simulink model "Sim7_test_var_load"  (R2018a)
settings: Solver=ode1  StartTime=0.0  StopTime=10  FixedStep=Time_Step  MaxStep=1e-4  RelTol=1e-3
undefined symbols (not defined in the file): Bxx_GenericVoltageSource, Lg, Rg, Source_Lib, Theta0, Time_Step, Ug, Un, V0, VSC01_id0
libraries: powerlib x29, Control_Lib x5, simulink x4
(part 1 of 2)
settings Model: Creator=Frederic_Colas  LastModifiedBy=fcolas
settings OptimizationCC: LifeSpan=inf
settings DebuggingCC: UnconnectedInputMsg=none  UnconnectedOutputMsg=none  UnconnectedLineMsg=none  SFExecutionAtInitializationDiag=none
settings HardwareCC: ProdBitPerSizeT=32  ProdBitPerPtrDiffT=32  ProdWordSize=32  ProdHWDeviceType=Specified
settings CodeAppCC: StateflowObjectComments=on
settings SimscapeCC: SimscapeNormalizeSystem=off

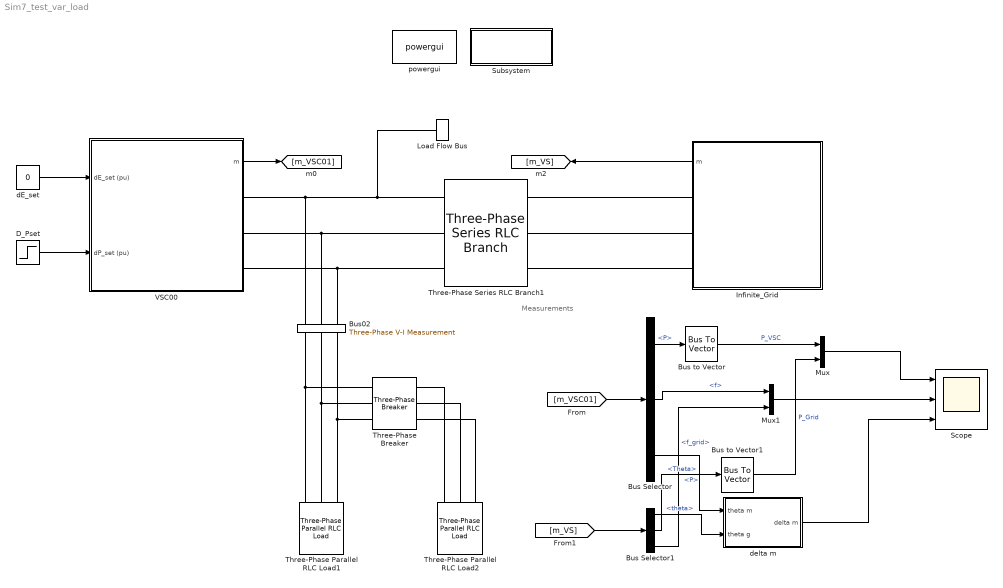
== system Sim7_test_var_load ==
  note: Measurements
  Bus Selector : BusSelector  OutputSignals=P,f,Theta.Theta
  Bus Selector1 : BusSelector  OutputSignals=Theta.theta,P,f_grid
  Bus to Vector : BusToVector
  Bus to Vector1 : BusToVector
  "Bus02 " : powerlib/Measurements/Three-Phase V-I Measurement  VoltageMeasurement=no  SetLabelV=off  LabelV=Vabc  Vpu=off  VpuLL=off  CurrentMeasurement=no  SetLabelI=off  LabelI=Iabc  Ipu=off  Pbase=100e6  Vbase=500e3  OutputType=Complex  PhasorSimulation=off  PSBequivalent=0
  D_Pset : Step  After=0  SampleTime=0
  Infinite_Grid : Subsystem  AncestorBlock=Source_Lib/Bxx_GenericVoltageSource  mask(GenericVoltageSource){SourceNature_str=INERTIAL, fn=50, Sn=1e9, Un=Un, LFpopup=Swing, P0=149805764.7076, Q0=1121677.2891, V0_pu=1, U0=20000, Theta0_deg=0, H_s=5, DroopOnOff=on, R_percent=4, TN=1, TD=2}
      mask prompts: SourceNature_str "Nature of the voltage source"; fn "Nominal frequency fn [Hz]"; Sn "Nominal apparent power Sn [VA]"; Un "Nominal voltage Un [V RMS Ph2Ph]"; P0 "Active power P0 [W]"; Q0 "Reactive power Q0 [VAR]"; V0_pu "Initial pu voltage V0_pu [pu]"; U0 "Initial voltage U0 [Vrms Ph2Ph]"; Theta0_deg "Initial angle (°)"; H_s "Inertia H [s]"; DroopOnOff "Frequency DROOP activation"; R_percent "Droop gain Kp [%]"; TN "Network time constant Lead [s]"; TD "Network time constant Lag [s]"
      mask init:
      | % Update Name of LF bus for internal purpose
      | NameStr = [get_param(gcb,'Name')];% '_LF'];
      | set_param([gcb '/Load Flow Bus'],'ID',NameStr);  
      | 
      | % Base specification
      | fb = fn;                % [Hz] base frequency
      | Sb = Sn;                % [VA] base power
      | Ub = Un;                % [V] base ph2ph voltage
      | Vb = Un/sqrt(3);        % [V] base ph2N voltage
      | Ib = Sb/(3*Vb);         % [A] base current
      | Zb = Vb*Ib;             % [Ohm] base impedance
      | 
      | % Set the frequency droop gain
      | R = R_percent / 100;
      | 
      | %Initialize correctly the LoadFlow bus parameters connected to PCC
      |     VLF = V0_pu;
      |     ThetaLF = Theta0_deg;
      |     if (LFpopup == 'PQ')
      |         VLF = 1;
      |         ThetaLF = 0;
      |     elseif (LFpopup == 'PV')
      |         VLF = V0_pu;
      |         ThetaLF = 0;        
      |     end
      |     set_param([gcb '/Load Flow Bus'],'Vref',num2str(VLF),'Vangle',num2str(ThetaLF));
      | 
      | 
      | % Update mask display:
      | % mo = get_param(gcb,'MaskObject');
      mask TypeOptions SourceNature_str: INFINITE | INERTIAL
      mask Callback SourceNature_str:
      | % Get the mask parameter values. This is a cell
      | %   array of character vectors.
      | maskStr = get_param(gcb,'SourceNature_str');
      | p=Simulink.Mask.get(gcb);
      | 
      | % The pop-up menu is the first mask parameter.
      | %   Check the value selected in the pop-up
      | if strcmp(maskStr,'INFINITE')
      |    p.getParameter('H_s').Visible='off';
      |    p.getParameter('DroopOnOff').Visible='off';
      |    DroopOnOff = 'off';
      |    p.getParameter('R_percent').Visible='off';
      |    p.getParameter('TN').Visible='off';
      |    p.getParameter('TD').Visible='off';
      |    set_param([gcb '/SourceNature'],'Value','1')
      | else
      |    p.getParameter('H_s').Visible='on';
      |    p.getParameter('DroopOnOff').Visible='on';
      |    DroopOnOff = 'on';
      |    p.getParameter('R_percent').Visible='on';
      |    p.getParameter('TN').Visible='on';
      |    p.getParameter('TD').Visible='on';
      |    set_param([gcb '/SourceNature'],'Value','2')
      | end
      mask TypeOptions LFpopup: Swing | PQ | PV
      mask Callback LFpopup:
      | % Get the mask parameter values. This is a cell
      | %   array of character vectors.
      | maskStr = get_param(gcb,'LFpopup');
      | p=Simulink.Mask.get(gcb);
      | 
      | % The pop-up menu is the first mask parameter.
      | %   Check the value selected in the pop-up
      | if strcmp(maskStr,'Swing'),
      | 
      |     % Set the visibility of both parameters on when
      |     %   User-defined is selected in the pop-up.
      |     p.getParameter('P0').Enabled='off';
      |     p.getParameter('Q0').Enabled='off';
      |     p.getParameter('V0_pu').Enabled='on';
      |     p.getParameter('U0').Enabled='off';
      |     p.getParameter('Theta0_deg').Enabled='off';
      |     set_param([gcb '/Source_For_LF'],'BusType','swing');
      | 
      | elseif strcmp(maskStr,'PQ'),
      | 
      |     % Set the visibility of both parameters on when
      |     %   User-defined is selected in the pop-up.
      |     p.getParameter('P0').Enabled='on';
      |     p.getParameter('Q0').Enabled='on';
      |     p.getParameter('V0_pu').Enabled='off';
      |     p.getParameter('U0').Enabled='off';
      |     p.getParameter('Theta0_deg').Enabled='off';
      |     set_param([gcb '/Source_For_LF'],'BusType','PQ');
      | 
      |     % Turn off the visibility of the Value field
      |     %   when User-defined is not selected.
      | else
      | 
      |     % Set the visibility of both parameters on when
      |     %   User-defined is selected in the pop-up.
      |     p.getParameter('P0').Enabled='on';
      |     p.getParameter('Q0').Enabled='off';
      |     p.getParameter('V0_pu').Enabled='on';
      |     p.getParameter('U0').Enabled='off';
      |     p.getParameter('Theta0_deg').Enabled='off';
      |     set_param([gcb '/Source_For_LF'],'BusType','PV');
      | 
      | end
      mask Callback DroopOnOff:
      | % Get the mask parameter values. This is a cell
      | %   array of character vectors.
      | maskStr = get_param(gcb,'DroopOnOff');
      | p=Simulink.Mask.get(gcb);
      | 
      | if strcmp(maskStr,'on'),
      |     p.getParameter('R_percent').Enabled='on';
      | else
      |     p.getParameter('R_percent').Enabled='off';
      | end
      mask DialogControl Container2 Prompt: Nominal specification (for base definition)
      mask DialogControl Container3 Prompt: Loadflow specification
      mask DialogControl InertialConfig Prompt: Inertial source configuration
  Load Flow Bus : powerlib/Measurements/Load Flow Bus  LConnTagsString=a  Phases=single  Connectors=on one side  ID=BUS_1  Vbase=Un  Vref=1  Vangle=0  VLF=0.9992  VLFb=1  VLFc=1  angleLF=-0.4292  angleLFb=0  angleLFc=0
  Mux : Mux  Inputs=2
  Mux1 : Mux  Inputs=2
  Scope : Scope  NumInputPorts=3
  Subsystem : Subsystem
      settings: OpenFcn=LoadFlow_VSC
      mask Display: color('blue'),disp('Update Loadflow')
  Three-Phase Parallel RLC Load1 : powerlib/Elements/Three-Phase Parallel RLC Load  LConnTagsString=A|B|C  Configuration=Y (grounded)  NominalVoltage=Ug  Vabc=[1e3 1e3 1e3]  Vabcp=[1e3 1e3 1e3]  NominalFrequency=fb  UnbalancedPower=off  ActivePower=300e6  InductivePower=0  CapacitivePower=0  Pabc=[10e3 9e3 11e3]  QLabc=[100 90 110]  QCabc=[100 90 110]  Pabcp=[10e3 9e3 11e3]  QLabcp=[100 90 110]  QCabcp=[100 90 110]  Measurements=None  LoadType=constant Z
  Three-Phase Parallel RLC Load2 : powerlib/Elements/Three-Phase Parallel RLC Load  LConnTagsString=A|B|C  Configuration=Y (grounded)  NominalVoltage=Ug  Vabc=[1e3 1e3 1e3]  Vabcp=[1e3 1e3 1e3]  NominalFrequency=fb  UnbalancedPower=off  ActivePower=500e6  InductivePower=0  CapacitivePower=0  Pabc=[10e3 9e3 11e3]  QLabc=[100 90 110]  QCabc=[100 90 110]  Pabcp=[10e3 9e3 11e3]  QLabcp=[100 90 110]  QCabcp=[100 90 110]  Measurements=None  LoadType=constant Z
  Three-Phase Series RLC Branch1 : powerlib/Elements/Three-Phase Series RLC Branch  LConnTagsString=A|B|C  RConnTagsString=A|B|C  BranchType=RL  Resistance=Rg  Inductance=Lg  Capacitance=1e-6  Measurements=None
  Three-Phase Breaker : powerlib/Elements/Three-Phase Breaker  InitialState=open  SwitchA=on  SwitchB=on  SwitchC=on  SwitchTimes=0.5  External=off  BreakerResistance=0.01  SnubberResistance=1e6  SnubberCapacitance=inf  Measurements=None
  VSC00 : Subsystem  mask(VSC){fn=50, Sn=1000e6, Pn=1000e6, Udcn=640e3, Time_Step=Time_Step, Un1=320e3, Un2=Ug, Rt_pu=0.005, Lt_pu=0.15, Lm_pu=500, Rm_pu=500, Tr_PLL=10, Val_Freq_Support=off, R_percent=4, Rv=0.09, W_TVR=60, I_max_VI_pu=1.2, DX_DR=5, Val_Mod_H=off, I_max_pu=1.25, Tr_I_max=200, Advanced=off, gainpopup=With Inertia, f_Inertia_Less=5/(2*pi), zeta_Inertia_Less=1, Param_Inertia=PI, H_GFo=5, zeta_GFo=0.7, LFpopup=PQ, P0=0.15, Q0=2.3716e-08, V0=0.99922, Theta0=-0.42918}
      mask prompts: fn "Nominal Frequency (Hz)"; Sn "Nominal Apparent Power (VA)"; Pn "Nominal Power (W)"; Udcn "Nominal DC Voltage (V)"; Time_Step "Sample Time (s)"; Un1 "VSC side Nominal Ph-Ph Voltage (V)"; Un2 "Grid side Nominal Ph-Ph Voltage (V)"; Rt_pu "R (pu)"; Lt_pu "L (pu)"; Lm_pu "Rm (pu)"; Rm_pu "Lm (pu)"; Tr_PLL "Time response (ms)"; Val_Freq_Support "Frequency Support"; R_percent "Droop Gain (%)"; Rv "Damping Resistance (Rv)"; W_TVR "Dr filter"; I_max_VI_pu "Current Threshold (pu)"; Val_Mod_H "Inertia Modulation"; I_max_pu "I max (pu)"; Tr_I_max "Current Loop time response (ms)"; gainpopup "Strategy"; f_Inertia_Less "Bandwidth (Hz)"; zeta_Inertia_Less "Damping"; H_GFo "Inertia H (s)"; zeta_GFo "Damping Ratio"; P0 "Initial Active Power (pu)"; Q0 "Initial Reactive Power (pu)"; V0 "Initial Voltage (pu)"; Theta0 "Initial Angle (°)"
      mask init:
      | % Update Name of LF bus for internal purpose
      |     %NameStr = [get_param(gcb,'Name')];% '_LF'];
      |     %set_param([gcb '/Load Flow Bus'],'ID',NameStr);    
      |     
      | % Base values
      |     fb = fn;
      |     Pb = Pn;
      |     cos_phi_n = Pn/Sn;
      |     Sb = Pb/cos_phi_n;
      |     Vn1 = Un1/sqrt(3);
      |     Vb1 = Vn1;
      |     Vn2 = Un2/sqrt(3);
      |     Vb2 = Vn2;
      |     Ib1 = Sb / 3*Vb1;
      |     Ib2 = Sb / (3*Vb2);
      |     wb = 2*pi*fb;
      |   
      | % PLL derivation of the parameters
      |     wn_PLL=5/Tr_PLL;
      |     zeta_PLL = 1;
      |     Kp_PLL_pu = 2*zeta_PLL*wn_PLL/wb;
      |     Ki_PLL_pu = wn_PLL^2/wb;
      |     
      | % Grid-Forming control tuning
      |     % Inertia Less
      |     wn_Inertia_Less = 2*pi*f_Inertia_Less;
      |     Ki_Inertia_Less = Lt_pu*wn_Inertia_Less^2/wb;
      |     Kp_Inertia_Less = 2*zeta_Inertia_Less*wn_Inertia_Less*Lt_pu/wb;
      |     
      |     % With Inertia
      |     Kc = 1/(Lt_pu);
      |     kp_GFo = zeta_GFo*sqrt(2/(H_GFo*wb*Kc));
      |     kd = 2*H_GFo*kp_GFo*Kc*wb;
      | 
      | % Virtual Impedance tuning
      |     X_VI = roots([1/DX_DR^2+1 2*Lt_pu Lt_pu^2-1/I_max_VI_pu^2]);
      |     X_VI = max(X_VI);
      |     Kp_Rvi_pu = X_VI/(DX_DR*(I_max_VI_pu-1)); 
      |     
      | % Set the chosen strategy
      |     if (gainpopup == 1)
      |         Chosen_Strategy = 1;
      |     elseif (gainpopup == 2)
      |         if (Param_Inertia == 1)
      |             Chosen_Strategy = 2;
      |         elseif (Param_Inertia == 2)
      |             Chosen_Strategy = 3;
      |         end
      |     end
      |     
      | % Set the frequency droop gain
      |     R = R_percent / 100;
      | 
      | % Compute the delay compensation between control and power parts
      |     if (Time_Step == -1)
      |         Solver_Time_Step = 0;
      |     else
      |         Solver_Time_Step = Time_Step;
      |     end
      | 
      | % Compute Initial Voltage of VSC 
      | %   from steady-state output transformer model and Loadflow result
      |     
      |     %Initialize correctly the LoadFlow bus parameters connected to PCC
      |     VLF = V0;
      |     ThetaLF = Theta0;
      |     %if (LFpopup == 'PQ')
      |     %    VLF = 1;
      |     %    ThetaLF = 0;
      |     %elseif (LFpopup == 'PV')
      |     %%    VLF = V0;
      |     %    ThetaLF = 0;        
      |     %end
      |     %set_param([gcb '/Load Flow Bus'],'Vref',num2str(VLF),'Vangle',num2str(ThetaLF));
      |     
      |     R1_pu = Rt_pu/2;
      |     L1_pu = Lt_pu/2;
      |     R2_pu = Rt_pu/2;
      |     L2_pu = Lt_pu/2;
      |     X1_pu = L1_pu;
      |     X2_pu = L2_pu;
      |     Xm_pu = Lm_pu;
      |     
      |     Zm_pu = 1/(1/Rm_pu+1/(1i*Xm_pu));
      | 
      |     S0=P0+1i*Q0;
      |     I2 = conj(S0)/(V0);
      | 
      |     Vm = (R2_pu+1i*X2_pu)*I2 + V0;
      |     Im = Vm/Zm_pu;
      | 
      |     I1 = I2 + Im;
      |     V1 = (R1_pu+1i*X1_pu) * I1 + Vm;
      | 
      |     Vvsc0 = abs(V1);
      |     Theta_vsc0 = angle(V1) * 180/pi+Theta0;
      |     
      |     Va0 = Vvsc0*sqrt(2)*Vb1*sin(Theta_vsc0*pi/180);
      |     Vb0 = Vvsc0*sqrt(2)*Vb1*sin(Theta_vsc0*pi/180-2*pi/3);
      |     Vc0 = Vvsc0*sqrt(2)*Vb1*sin(Theta_vsc0*pi/180+2*pi/3);
      |     
      | % Generate string to display LF results on Mask
      |     %str_tmp = fprintf("Vvsc0 = %d, Theta_vsc0 = %d°",Vvsc0,Theta_vsc0);
      |     mo = get_param(gcb,'MaskObject');
      |     mo.getDialogControl('LF_vsc_str').Prompt = ['V0 = ', num2str(Vvsc0),' pu, Angle = ', num2str(Theta_vsc0),'°'];
      |     mo.getDialogControl('LF_pcc_str').Prompt = ['V0 = ', num2str(V0),' pu, Angle = ', num2str(Theta0),'°'];
      |     mo.getDialogControl('LF_pcc_Power_str').Prompt = ['P0 = ', num2str(P0),' pu, Q0 = ', num2str(Q0),' pu'];
      |     %set_param([gcb],'LF_str',str_tmp);
      settings: OpenFcn=|
      | NameStr = get_param(gcb,'Name');
      | open_system(gcbh, 'Mask');
      | 
      | h2AllOpenDlgs = DAStudio.ToolRoot.getOpenDialogs;
      | 
      | for i=1:length(h2AllOpenDlgs)
      |     try
      |          %disp(h2AllOpenDlgs(i).getSource.getBlock.Name);
      |         Dialog_block_name = h2AllOpenDlgs(i).getSource.getBlock.Name;
      |          %strcmp(Dialog_block_name, NameStr),
      |         if (strcmp(h2AllOpenDlgs(i).getSource.getBlock.Name, NameStr))
      |             iPos = h2AllOpenDlgs(i).position;
      |             h2AllOpenDlgs(i).position = [iPos(1)   iPos(2)   iPos(3)*1.4   iPos(4)];
      |         end
      |     end
      | end
      mask Callback Advanced:
      | % Get the mask parameter values. This is a cell
      | %   array of character vectors.
      | maskStr = get_param(gcb,'Advanced');
      | p=Simulink.Mask.get(gcb);
      | 
      | % The pop-up menu is the first mask parameter.
      | %   Check the value selected in the pop-up
      | if strcmp(maskStr,'on'),
      | 
      |     % Set the visibility of both parameters on when
      |     %   User-defined is selected in the pop-up.
      |     p.getDialogControl('TVR').Visible='on';
      |     p.getDialogControl('TVI').Visible='on';
      |     %p.getDialogControl('LC_Filter').Visible='on';
      |     p.getDialogControl('Current_Sat').Visible='on';
      |     %p.getDialogControl('Param_Strat_3').Visible='off';
      | 
      | 
      | else
      | 
      |     % Set the visibility of both parameters on when
      |     %   User-defined is selected in the pop-up.
      |     p.getDialogControl('TVR').Visible='off';
      |     p.getDialogControl('TVI').Visible='off';
      |     %p.getDialogControl('LC_Filter').Visible='off';
      |     p.getDialogControl('Current_Sat').Visible='off';
      |     %p.getDialogControl('Param_Strat_3').Visible='off';
      | 
      | end
      mask TypeOptions gainpopup: Inertia Less | With Inertia
      mask Callback gainpopup:
      | % Get the mask parameter values. This is a cell
      | %   array of character vectors.
      | maskStr = get_param(gcb,'gainpopup');
      | p=Simulink.Mask.get(gcb);
      | 
      | % The pop-up menu is the first mask parameter.
      | %   Check the value selected in the pop-up
      | if strcmp(maskStr,'Inertia Less'),
      | 
      |     % Set the visibility of both parameters on when
      |     %   User-defined is selected in the pop-up.
      |     p.getDialogControl('No_Inertia').Visible='on';
      |     p.getDialogControl('Inertia').Visible='off';
      |     %p.getDialogControl('Param_Strat_3').Visible='off';
      | 
      | 
      | elseif strcmp(maskStr,'With Inertia'),
      | 
      |     % Set the visibility of both parameters on when
      |     %   User-defined is selected in the pop-up.
      |     p.getDialogControl('No_Inertia').Visible='off';
      |     p.getDialogControl('Inertia').Visible='on';
      |     %p.getDialogControl('Param_Strat_3').Visible='off';
      | 
      | 
      |     % Turn off the visibility of the Value field
      |     %   when User-defined is not selected.
      | 
      | else
      | 
      |     % Set the visibility of both parameters on when
      |     %   User-defined is selected in the pop-up.
      |     p.getDialogControl('No_Inertia').Visible='off';
      |     p.getDialogControl('Inertia').Visible='off';
      |     %p.getDialogControl('Param_Strat_3').Visible='off';
      | 
      | end
      mask TypeOptions Param_Inertia: VSM | PI
      mask TypeOptions LFpopup: Swing | PQ | PV
      mask Callback LFpopup:
      | % Get the mask parameter values. This is a cell
      | %   array of character vectors.
      | maskStr = get_param(gcb,'LFpopup');
      | p=Simulink.Mask.get(gcb);
      | 
      | % The pop-up menu is the first mask parameter.
      | %   Check the value selected in the pop-up
      | if strcmp(maskStr,'Swing'),
      | 
      |     % Set the visibility of both parameters on when
      |     %   User-defined is selected in the pop-up.
      |     p.getParameter('P0').Visible='off';
      |     p.getParameter('Q0').Visible='off';
      |     p.getParameter('V0').Visible='on';
      |     p.getParameter('Theta0').Visible='on';
      |     set_param([gcb '/Source_For_LF'],'BusType','swing');
      | 
      | elseif strcmp(maskStr,'PQ'),
      | 
      |     % Set the visibility of both parameters on when
      |     %   User-defined is selected in the pop-up.
      |     p.getParameter('P0').Visible='on';
      |     p.getParameter('Q0').Visible='on';
      |     p.getParameter('V0').Visible='off';
      |     p.getParameter('Theta0').Visible='off';
      |     set_param([gcb '/Source_For_LF'],'BusType','PQ');
      | 
      |     % Turn off the visibility of the Value field
      |     %   when User-defined is not selected.
      | else
      | 
      |     % Set the visibility of both parameters on when
      |     %   User-defined is selected in the pop-up.
      |     p.getParameter('P0').Visible='on';
      |     p.getParameter('Q0').Visible='off';
      |     p.getParameter('V0').Visible='on';
      |     p.getParameter('Theta0').Visible='off';
      |     set_param([gcb '/Source_For_LF'],'BusType','PV');
      | 
      | end
      mask DialogControl Nominal_Param Prompt: Nominal Value
      mask DialogControl Container20 Prompt: Passive Components
      mask DialogControl Control_Param Prompt: Control Parameter
      mask DialogControl Container13 Prompt: PLL
      mask DialogControl Container14 Prompt: Frequency Support
      mask DialogControl TVR Prompt: Transient Virtual Resistor
      mask DialogControl TVI Prompt: Virtual Impedance
      mask DialogControl Current_Sat Prompt: Current Limitation
      mask DialogControl Container18 Prompt: Control Strategy
      mask DialogControl LF_Param Prompt: Loadflow
      mask DialogControl Control4 Prompt: Initial Operating Point
      mask DialogControl Container24 Prompt: VSC side
      mask DialogControl LF_vsc_str Prompt: V0 = 1.0004 pu, Angle = 0.869°
      mask DialogControl Container25 Prompt: PCC
      mask DialogControl LF_pcc_str Prompt: V0 = 0.99922 pu, Angle = -0.42918°
      mask DialogControl LF_pcc_Power_str Prompt: P0 = 0.15 pu, Q0 = 2.3716e-08 pu
      mask DialogControl UpdateLoadflow Prompt: Update Loadflow
      mask DialogControl UpdateLoadflow Callback: LoadFlow_VSC
      mask Display:
      | x1=0.05;
      | y1=0.2;
      | %
      | plot([0.5 0.5]+x1,[0.97,0.8]-y1)
      | plot([0.5 0.32]+x1,[0.80 0.71]-y1)
      | plot([0.32 0.32]+x1,[0.80 0.52]-y1)
      | plot([0.32 0.5]+x1,[0.62 0.52]-y1)
      | plot([0.5 0.5]+x1,[0.52 0.35]-y1)
      | plot([0.45 0.5 0.43]+x1,[0.59 0.52 0.51]-y1)
      | %
      | plot([0.28 0.28]+x1,[0.74 0.58]-y1)
      | plot([0.28 0.20]+x1,[0.66 0.66]-y1)
      | %
      | plot([0.5 0.63]+x1,[0.84 0.84]-y1)
      | plot([0.63 0.63]+x1,[0.84 0.72]-y1)
      | plot([0.63 0.59]+x1,[0.72 0.65]-y1)
      | plot([0.63 0.67]+x1,[0.72 0.65]-y1)
      | plot([0.59 0.67]+x1,[0.65 0.65]-y1)
      | plot([0.63 0.63]+x1,[0.65 0.47]-y1)
      | plot([0.5 0.63]+x1,[0.47 0.47]-y1)
      | plot([0.58 0.67]+x1,[0.72 0.72]-y1)
      | %
      | color('blue')
      | text(0.3,0.10,'L-Filter GFo')
      | port_label('input',1,'dE_set (pu)');
      | port_label('input',2,'dP_set (pu)');
      | port_label('output',1,'m');
      | port_label('rconn',1,'A');
      | port_label('rconn',2,'B');
      | port_label('rconn',3,'C');
  dE_set : Constant  Value=0
  delta m : Subsystem
  powergui : powerlib/powergui  Priority=1  SimulationMode=Discrete  SampleTime=Time_Step  frequency=60  Iterations=50  frequencyindice=50  Pbase=1000000000  ErrMax=1e-6  UnitsV=kV  UnitsW=MW  buscounter=0  FunctionMessages=off  echomessages=off  EnableUseOfTLC=off  CurrentSourceSwitches=off  DisableSnubberDevices=off  DisableRonSwitches=off  DisableVfSwitches=off  DisplayEquations=off  AutomaticDiscreteSolvers=off  SolverType=Tustin/Backward Euler (TBE)  Interpol=off  ExternalGateDelay=off  methode=off  Ts=100  x0status=blocks  SPID=on  SwTol=0  HookPort=off  NonlinearTolerance=1e-4  nMaxIteration=100  ContinueOnMaxIteration=off  RestoreLinks=warning  ResistiveCurrentMeasurement=off  Frange=[0:2:500]  Ylog=off  Xlog=on  ShowGrid=off  save=off  variable=ZData  structure=0  ZoomFFT=off  StartTime=0.0  cycles=1  DisplayStyle=1  fundamental=60  FreqAxis=off  MaxFrequency=1000  frequencyindicesteady=1  RmsSteady=1  display=off
  wires:
  dE_set/1 -> VSC00/1(dE_set (pu))
  D_Pset/1 -> VSC00/2(dP_set (pu))
  VSC00/1(m) -> [m_VSC01]
  Infinite_Grid/1(m) -> [m_VS]
  Bus Selector1/1 -> delta m/2(theta g)  "<theta>"
  Bus Selector/2 -> Mux1/1  "<f>"
  [m_VSC01] -> Bus Selector/1
  [m_VS] -> Bus Selector1/1
  Bus Selector/3 -> delta m/1(theta m)  "<Theta>"
  Bus Selector1/2 -> Bus to Vector1/1  "<P>"
  Mux/1 -> Scope/1
  Mux1/1 -> Scope/2
  Bus Selector/1 -> Bus to Vector/1  "<P>"
  Bus Selector1/3 -> Mux1/2  "<f_grid>"
  Bus to Vector/1 -> Mux/1  "P_VSC"
  Bus to Vector1/1 -> Mux/2  "P_Grid"
  delta m/1(delta m) -> Scope/3
  connections:
  VSC00/RConn1 -- "Bus02 "/LConn3 -- Load Flow Bus/LConn1 -- Three-Phase Series RLC Branch1/LConn1
  VSC00/RConn3 -- "Bus02 "/LConn1 -- Three-Phase Series RLC Branch1/LConn3
  VSC00/RConn2 -- "Bus02 "/LConn2 -- Three-Phase Series RLC Branch1/LConn2
  Infinite_Grid/RConn1 -- Three-Phase Series RLC Branch1/RConn1
  Infinite_Grid/RConn2 -- Three-Phase Series RLC Branch1/RConn2
  Infinite_Grid/RConn3 -- Three-Phase Series RLC Branch1/RConn3
  Three-Phase Breaker/LConn2 -- Three-Phase Parallel RLC Load1/LConn2 -- "Bus02 "/RConn2
  Three-Phase Breaker/LConn1 -- Three-Phase Parallel RLC Load1/LConn1 -- "Bus02 "/RConn3
  Three-Phase Breaker/LConn3 -- Three-Phase Parallel RLC Load1/LConn3 -- "Bus02 "/RConn1
  Three-Phase Parallel RLC Load2/LConn3 -- Three-Phase Breaker/RConn3
  Three-Phase Parallel RLC Load2/LConn2 -- Three-Phase Breaker/RConn2
  Three-Phase Breaker/RConn1 -- Three-Phase Parallel RLC Load2/LConn1

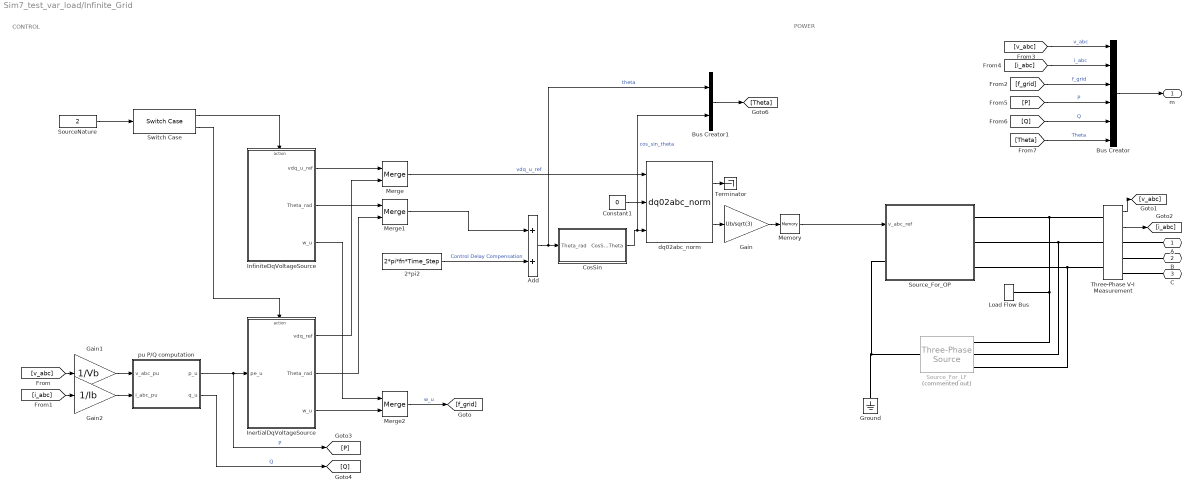
== system Sim7_test_var_load/Infinite_Grid ==
  note: POWER
  note: CONTROL
  " pu P/Q computation" : Subsystem  DialogController=POWERSYS.PowerSysDialog
  2*pi2 : Constant  Value=2*pi*fn*Time_Step
  Add : Sum
  Bus Creator : BusCreator  Inputs=6
  Bus Creator1 : BusCreator  Inputs=2
  Constant1 : Constant  Value=0
  CosSin : Subsystem
  Gain : Gain  Gain=Ub/sqrt(3)
  Gain1 : Gain  Gain=1/Vb
  Gain2 : Gain  Gain=1/Ib
  Ground : powerlib/Elements/Ground  LConnTagsString=a
  InertialDqVoltageSource : Subsystem  TreatAsAtomicUnit=on
  InfiniteDqVoltageSource : Subsystem  TreatAsAtomicUnit=on
  Load Flow Bus : powerlib/Measurements/Load Flow Bus  LConnTagsString=a  Phases=single  Connectors=on one side  ID=Infinite_Grid  Vbase=Un  Vref=1  Vangle=0  VLF=1  VLFb=1  VLFc=1  angleLF=0  angleLFb=0  angleLFc=0
  Memory : Memory
  Merge : Merge
  Merge1 : Merge
  Merge2 : Merge
  SourceNature : Constant  Value=2
  Source_For_LF : powerlib/Electrical Sources/Three-Phase Source  Commented=on  InternalConnection=Yn  VoltagePhases=off  Voltage=(400000)*1  PhaseAngle=0  Voltage_phases=[25e3 25e3 25e3]/sqrt(3)  PhaseAngles_phases=[0 -120 +120]  Frequency=fb  NonIdealSource=off  SpecifyImpedance=off  Resistance=0  Inductance=0  ShortCircuitLevel=100e6  BaseVoltage=Un  XRratio=7  BusType=swing  Pref=P0  Qref=Q0  Prefabc=[10e3, 10e3, 10e3]  Qrefabc=[0, 0, 0]  Qmin=-inf  Qmax=inf
  Source_For_OP : Subsystem
  Switch Case : SwitchCase  CaseConditions={1, 2}  ShowDefaultCase=off
  Terminator : Terminator
  Three-Phase V-I Measurement : powerlib/Measurements/Three-Phase V-I Measurement  VoltageMeasurement=phase-to-ground  SetLabelV=off  LabelV=v_abc  Vpu=off  VpuLL=off  CurrentMeasurement=yes  SetLabelI=off  LabelI=i_abc  Ipu=off  Pbase=100e6  Vbase=500e3  OutputType=Complex  PhasorSimulation=off  PSBequivalent=0
  dq02abc_norm : Control_Lib/dq02abc_norm  referenceAxisMode=Reference axis at 90 degrees behind phase_a  baseUpdateGain=sqrt(3)
      settings: SourceProductName=VSC_Lib
  A : PMIOPort  Side=Right
  B : PMIOPort  Port=2  Side=Right
  C : PMIOPort  Port=3  Side=Right
  m : Outport  VectorParamsAs1DForOutWhenUnconnected=off
  wires:
  [Q] -> Bus Creator/5  "Q"
  [P] -> Bus Creator/4  "P"
  Three-Phase V-I Measurement/2 -> [i_abc]
  Three-Phase V-I Measurement/1 -> [v_abc]
  Bus Creator/1 -> m/1
  Merge2/1 -> [f_grid]  "w_u"
  InfiniteDqVoltageSource/3(w_u) -> Merge2/1
  [f_grid] -> Bus Creator/3  "f_grid"
  [i_abc] -> Bus Creator/2  "i_abc"
  [v_abc] -> Bus Creator/1  "v_abc"
  InertialDqVoltageSource/3(w_u) -> Merge2/2
  2*pi2/1 -> Add/2  "Control Delay Compensation"
  Merge1/1 -> Add/1
  Add/1 -> Bus Creator1/1, CosSin/1(Theta_rad)  "theta"
  Memory/1 -> Source_For_OP/1(v_abc_ref)
  " pu P/Q computation"/1(p_u) -> InertialDqVoltageSource/1(pe_u), [P]  "P"
  " pu P/Q computation"/2(q_u) -> [Q]  "Q"
  CosSin/1(CosSinTheta) -> Bus Creator1/2, dq02abc_norm/3  "cos_sin_theta"
  Gain2/1 -> " pu P/Q computation"/2(i_abc_pu)
  Gain1/1 -> " pu P/Q computation"/1(v_abc_pu)
  [i_abc] -> Gain2/1
  [v_abc] -> Gain1/1
  Switch Case/2 -> InertialDqVoltageSource/Action
  InertialDqVoltageSource/2(Theta_rad) -> Merge1/2
  InfiniteDqVoltageSource/2(Theta_rad) -> Merge1/1
  Merge/1 -> dq02abc_norm/1  "vdq_u_ref"
  InertialDqVoltageSource/1(vdq_ref) -> Merge/2
  InfiniteDqVoltageSource/1(vdq_u_ref) -> Merge/1
  Switch Case/1 -> InfiniteDqVoltageSource/Action
  SourceNature/1 -> Switch Case/1
  Gain/1 -> Memory/1
  dq02abc_norm/1 -> Terminator/1
  Constant1/1 -> dq02abc_norm/2
  dq02abc_norm/2 -> Gain/1
  Bus Creator1/1 -> [Theta]
  [Theta] -> Bus Creator/6  "Theta"
  connections:
  Three-Phase V-I Measurement/RConn3 -- C/RConn1
  Three-Phase V-I Measurement/RConn2 -- B/RConn1
  Three-Phase V-I Measurement/RConn1 -- A/RConn1
  Three-Phase V-I Measurement/LConn1 -- Load Flow Bus/LConn1 -- Source_For_LF/RConn1 -- Source_For_OP/RConn1
  Source_For_OP/RConn3 -- Three-Phase V-I Measurement/LConn3 -- Source_For_LF/RConn3
  Source_For_LF/LConn1 -- Ground/LConn1 -- Source_For_OP/LConn1
  Source_For_OP/RConn2 -- Three-Phase V-I Measurement/LConn2 -- Source_For_LF/RConn2

== system Sim7_test_var_load/Subsystem ==

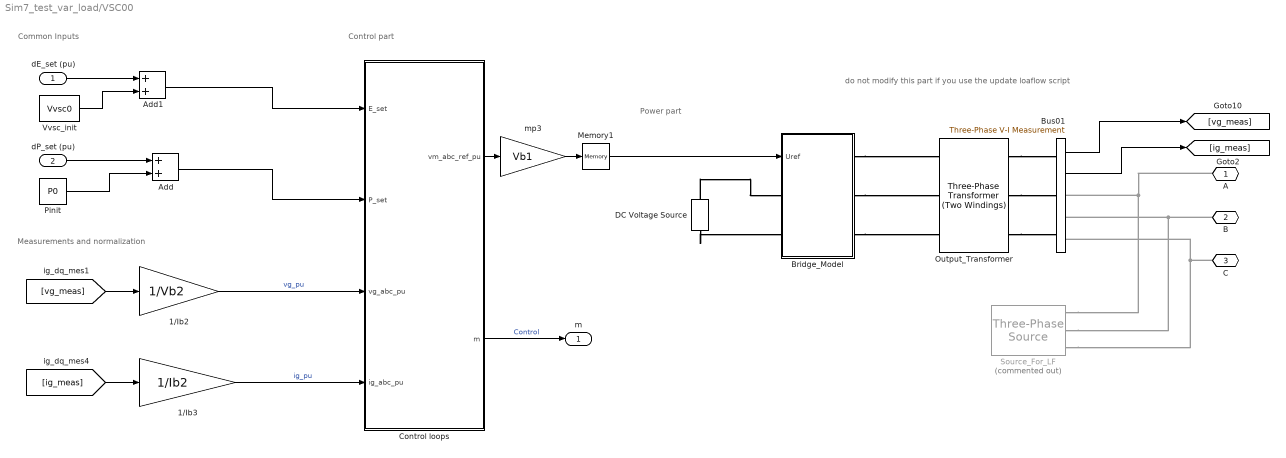
== system Sim7_test_var_load/VSC00 ==
  note: do not modify this part if you use the update loaflow script
  note: Common Inputs
  note: Power part
  note: Measurements and normalization
  note: Control part
  dE_set (pu) : Inport
  dP_set (pu) : Inport  Port=2
  1/Ib2 : Gain  Gain=1/Vb2
  1/Ib3 : Gain  Gain=1/Ib2
  Add : Sum
  Add1 : Sum
  Bridge_Model : Subsystem
  Bus01 : powerlib/Measurements/Three-Phase V-I Measurement  VoltageMeasurement=phase-to-ground  SetLabelV=off  LabelV=Vabc  Vpu=off  VpuLL=off  CurrentMeasurement=yes  SetLabelI=off  LabelI=Iabc  Ipu=off  Pbase=100e6  Vbase=500e3  OutputType=Complex  PhasorSimulation=off  PSBequivalent=0
  Control loops : Subsystem
  DC Voltage Source : powerlib/Electrical Sources/DC Voltage Source  Amplitude=Udcn  Measurements=Voltage
  Memory1 : Memory  InitialCondition=[Va0 Vb0 Vc0]
  Output_Transformer : powerlib/Elements/Three-Phase Transformer (Two Windings)  Winding1Connection=Yg  Winding2Connection=Yg  CoreType=Three single-phase transformers  SetSaturation=off  Hysteresis=off  DataFile='hysteresis'  SetInitialFlux=off  Measurements=None  UNITS=pu  NominalPower=[Sn , fb]  Winding1=[Un1 , Rt_pu/2 , Lt_pu/2]  Winding2=[Un2 , Rt_pu/2 , Lt_pu/2]  Rm=Rm_pu  Lm=Lm_pu  L0=0.5  Saturation=[ 0,0 ; 0.0024,1.2 ; 1.0,1.52 ]  InitialFluxes=[ 0.8 , -0.8 , 0.7 ]  BreakLoop=off  DiscreteSolver=Trapezoidal iterative  DataType=off  TransfoNumber=1
  Pinit : Constant  Value=P0
  Source_For_LF : powerlib/Electrical Sources/Three-Phase Source  Commented=on  InternalConnection=Yg  VoltagePhases=off  Voltage=(400000)*1.00139  PhaseAngle=0.85782  Voltage_phases=[25e3 25e3 25e3]/sqrt(3)  PhaseAngles_phases=[0 -120 +120]  Frequency=fb  NonIdealSource=off  SpecifyImpedance=off  Resistance=0  Inductance=0  ShortCircuitLevel=100e6  BaseVoltage=Un  XRratio=7  BusType=PQ  Pref=P0*Sb  Qref=Q0*Sb  Prefabc=[10e3, 10e3, 10e3]  Qrefabc=[0, 0, 0]  Qmin=-inf  Qmax=inf
  Vvsc_init : Constant  Value=Vvsc0
  mp3 : Gain  Gain=Vb1
  A : PMIOPort  Side=Right
  B : PMIOPort  Port=2  Side=Right
  C : PMIOPort  Port=3  Side=Right
  m : Outport  VectorParamsAs1DForOutWhenUnconnected=off
  wires:
  Add/1 -> Control loops/2(P_set)
  Control loops/2(m) -> m/1  "Control"
  mp3/1 -> Memory1/1
  1/Ib3/1 -> Control loops/4(ig_abc_pu)  "ig_pu"
  1/Ib2/1 -> Control loops/3(vg_abc_pu)  "vg_pu"
  [vg_meas] -> 1/Ib2/1
  Control loops/1(vm_abc_ref_pu) -> mp3/1
  Add1/1 -> Control loops/1(E_set)
  Memory1/1 -> Bridge_Model/1(Uref)
  dP_set (pu)/1 -> Add/1
  Pinit/1 -> Add/2
  Vvsc_init/1 -> Add1/2
  Bus01/1 -> [vg_meas]
  dE_set (pu)/1 -> Add1/1
  Bus01/2 -> [ig_meas]
  [ig_meas] -> 1/Ib3/1
  connections:
  DC Voltage Source/LConn1 -- Bridge_Model/LConn2
  Output_Transformer/RConn1 -- Bus01/LConn1
  Output_Transformer/RConn2 -- Bus01/LConn2
  DC Voltage Source/RConn1 -- Bridge_Model/LConn1
  Output_Transformer/RConn3 -- Bus01/LConn3
  Source_For_LF/RConn2 -- B/RConn1 -- Bus01/RConn2
  Bridge_Model/RConn1 -- Output_Transformer/LConn1
  Bridge_Model/RConn2 -- Output_Transformer/LConn2
  Bridge_Model/RConn3 -- Output_Transformer/LConn3
  Source_For_LF/RConn1 -- A/RConn1 -- Bus01/RConn1
  Source_For_LF/RConn3 -- C/RConn1 -- Bus01/RConn3

== system Sim7_test_var_load/delta m ==
  theta m : Inport
  theta g : Inport  Port=2
  Constant1 : Constant  Value=2*pi-1e-6
  Constant2 : Constant  Value=pi
  Math Function : Math  Operator=mod  SaturateOnIntegerOverflow=on
  Sum : Sum  Inputs=+-+
  Sum2 : Sum  Inputs=+-
  delta m : Outport
  wires:
  Sum2/1 -> delta m/1
  Math Function/1 -> Sum2/1
  theta g/1 -> Sum/2
  Sum/1 -> Math Function/1
  Constant1/1 -> Math Function/2
  theta m/1 -> Sum/1
  Constant2/1 -> Sum2/2, Sum/3

== system Sim7_test_var_load/Infinite_Grid/ pu P//Q computation ==
  v_abc_pu : Inport  PortDimensions=3
  i_abc_pu : Inport  Port=2  PortDimensions=3
  Demux : Demux  Outputs=3
      settings: DisplayOption=none
  Mux : Mux  Inputs=3
  Product1 : Product  InputSameDT=on  SaturateOnIntegerOverflow=on  OutDataTypeStr=Inherit: Same as first input
  Product3 : Product  InputSameDT=on  SaturateOnIntegerOverflow=on  OutDataTypeStr=Inherit: Same as first input
  Sum : Sum  Inputs=+-  InputSameDT=on  SaturateOnIntegerOverflow=on  OutDataTypeStr=Inherit: Same as first input
  Sum1 : Sum  Inputs=1  InputSameDT=on  SaturateOnIntegerOverflow=on  OutDataTypeStr=Inherit: Same as first input
  Sum4 : Sum  Inputs=1  InputSameDT=on  SaturateOnIntegerOverflow=on  OutDataTypeStr=Inherit: Same as first input
  Sum5 : Sum  Inputs=+-  InputSameDT=on  SaturateOnIntegerOverflow=on  OutDataTypeStr=Inherit: Same as first input
  Sum6 : Sum  Inputs=+-  InputSameDT=on  SaturateOnIntegerOverflow=on  OutDataTypeStr=Inherit: Same as first input
  pu->V : Gain  Gain=1/sqrt(3)  SaturateOnIntegerOverflow=on  OutDataTypeStr=Inherit: Same as input  ParamDataTypeStr=Inherit: Same as input
  pu->V1 : Gain  Gain=1/3  SaturateOnIntegerOverflow=on  OutDataTypeStr=Inherit: Same as input  ParamDataTypeStr=Inherit: Same as input
  pu->V2 : Gain  Gain=1/3  SaturateOnIntegerOverflow=on  OutDataTypeStr=Inherit: Same as input  ParamDataTypeStr=Inherit: Same as input
  p_u : Outport  VectorParamsAs1DForOutWhenUnconnected=off
  q_u : Outport  Port=2  VectorParamsAs1DForOutWhenUnconnected=off
  wires:
  pu->V/1 -> pu->V2/1  "Q"
  Mux/1 -> Product3/1
  Sum6/1 -> Mux/2
  Sum5/1 -> Mux/1
  Sum/1 -> Mux/3
  Demux/3 -> Sum6/1, Sum5/2
  Demux/2 -> Sum5/1, Sum/2
  Demux/1 -> Sum6/2, Sum/1
  Sum4/1 -> pu->V1/1
  i_abc_pu/1 -> Product3/2, Product1/2
  v_abc_pu/1 -> Demux/1, Product1/1
  Product1/1 -> Sum4/1
  Product3/1 -> Sum1/1
  Sum1/1 -> pu->V/1
  pu->V1/1 -> p_u/1
  pu->V2/1 -> q_u/1

== system Sim7_test_var_load/Infinite_Grid/CosSin ==
  Theta_rad : Inport
  Mux : Mux  Inputs=2
  Trigonometric Function : Trigonometry
  Trigonometric Function1 : Trigonometry  Operator=cos
  CosSinTheta : Outport  VectorParamsAs1DForOutWhenUnconnected=off
  wires:
  Trigonometric Function1/1 -> Mux/1
  Mux/1 -> CosSinTheta/1
  Trigonometric Function/1 -> Mux/2
  Theta_rad/1 -> Trigonometric Function1/1, Trigonometric Function/1

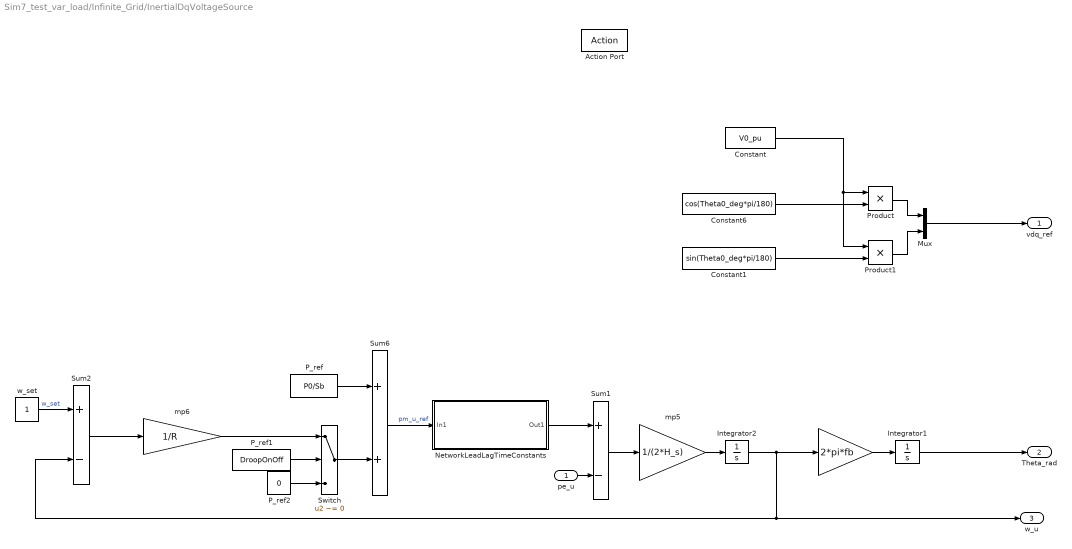
== system Sim7_test_var_load/Infinite_Grid/InertialDqVoltageSource ==
  pe_u : Inport
  Action Port : ActionPort
  " " : Gain  Gain=2*pi*fb
  Constant : Constant  Value=V0_pu
  Constant1 : Constant  Value=sin(Theta0_deg*pi/180)
  Constant6 : Constant  Value=cos(Theta0_deg*pi/180)
  Integrator1 : Integrator
  Integrator2 : Integrator  InitialCondition=1
  Mux : Mux  Inputs=2
  NetworkLeadLagTimeConstants : Subsystem
  P_ref : Constant  Value=P0/Sb
  P_ref1 : Constant  Value=DroopOnOff
  P_ref2 : Constant  Value=0
  Product : Product
  Product1 : Product
  Sum1 : Sum  Inputs=+-
  Sum2 : Sum  Inputs=+-
  Sum6 : Sum
  Switch : Switch  Criteria=u2 ~= 0
  mp5 : Gain  Gain=1/(2*H_s)
  mp6 : Gain  Gain=1/R
  w_set : Constant
  vdq_ref : Outport  VectorParamsAs1DForOutWhenUnconnected=off
  Theta_rad : Outport  Port=2  VectorParamsAs1DForOutWhenUnconnected=off
  w_u : Outport  Port=3  VectorParamsAs1DForOutWhenUnconnected=off
  wires:
  P_ref2/1 -> Switch/3
  mp6/1 -> Switch/1
  Switch/1 -> Sum6/2
  P_ref1/1 -> Switch/2
  NetworkLeadLagTimeConstants/1(Out1) -> Sum1/1
  Mux/1 -> vdq_ref/1
  Product/1 -> Mux/1
  Product1/1 -> Mux/2
  Constant/1 -> Product/1, Product1/1
  Constant6/1 -> Product/2
  Constant1/1 -> Product1/2
  Integrator1/1 -> Theta_rad/1
  w_set/1 -> Sum2/1  "w_set"
  pe_u/1 -> Sum1/2
  " "/1 -> Integrator1/1
  Sum1/1 -> mp5/1
  Sum2/1 -> mp6/1
  P_ref/1 -> Sum6/1
  Integrator2/1 -> " "/1, Sum2/2, w_u/1
  Sum6/1 -> NetworkLeadLagTimeConstants/1(In1)  "pm_u_ref"
  mp5/1 -> Integrator2/1

== system Sim7_test_var_load/Infinite_Grid/InfiniteDqVoltageSource ==
  Action Port : ActionPort
  Constant : Constant  Value=V0_pu
  Constant1 : Constant  Value=sin(Theta0_deg*pi/180)
  Constant4 : Constant
  Constant6 : Constant  Value=cos(Theta0_deg*pi/180)
  Gain : Gain  Gain=2*pi*fn
  Integrator : Integrator
  Mux : Mux  Inputs=2
  Product : Product
  Product1 : Product
  vdq_u_ref : Outport  VectorParamsAs1DForOutWhenUnconnected=off
  Theta_rad : Outport  Port=2  VectorParamsAs1DForOutWhenUnconnected=off
  w_u : Outport  Port=3  VectorParamsAs1DForOutWhenUnconnected=off
  wires:
  Constant4/1 -> Gain/1, w_u/1
  Mux/1 -> vdq_u_ref/1
  Integrator/1 -> Theta_rad/1
  Product1/1 -> Mux/2
  Constant/1 -> Product/1, Product1/1
  Constant6/1 -> Product/2
  Product/1 -> Mux/1
  Gain/1 -> Integrator/1
  Constant1/1 -> Product1/2

== system Sim7_test_var_load/Infinite_Grid/Source_For_OP ==
  v_abc_ref : Inport
  Controlled Voltage Source1 : powerlib/Electrical Sources/Controlled Voltage Source  Initialize=off  Source_Type=AC  Amplitude=V0*Ub*sqrt(2/3)*sin(Theta0)  Phase=(Theta0*180/pi)  Frequency=fb  Measurements=None
  Controlled Voltage Source2 : powerlib/Electrical Sources/Controlled Voltage Source  Initialize=off  Source_Type=AC  Amplitude=V0*Ub*sqrt(2/3)*sin(Theta0-2*pi/3)  Phase=(Theta0*180/pi)-120  Frequency=fb  Measurements=None
  Controlled Voltage Source3 : powerlib/Electrical Sources/Controlled Voltage Source  Initialize=off  Source_Type=AC  Amplitude=V0*Ub*sqrt(2/3)*sin(Theta0-4*pi/3)  Phase=(Theta0*180/pi)+120  Frequency=fb  Measurements=None
  Demux : Demux  Outputs=3
  Step : Step  Time=1e-9  SampleTime=0
  Subsystem3 : Subsystem
  Three-Phase Source1 : powerlib/Electrical Sources/Three-Phase Source  InternalConnection=Yn  VoltagePhases=off  Voltage=V0_pu*Ub  PhaseAngle=Theta0_deg  Voltage_phases=[25e3 25e3 25e3]/sqrt(3)  PhaseAngles_phases=[0 -120 +120]  Frequency=fb  NonIdealSource=off  SpecifyImpedance=off  Resistance=0.8929  Inductance=16.58e-3  ShortCircuitLevel=100e6  BaseVoltage=25e3  XRratio=7  BusType=swing  Pref=10e3  Qref=0  Prefabc=[10e3, 10e3, 10e3]  Qrefabc=[0, 0, 0]  Qmin=-inf  Qmax=inf
  A : PMIOPort  Side=Right
  B : PMIOPort  Port=2  Side=Right
  C : PMIOPort  Port=3  Side=Right
  N : PMIOPort  Port=4  Side=Left
  wires:
  Step/1 -> Subsystem3/1(switch)
  Demux/3 -> Controlled Voltage Source3/1
  Demux/1 -> Controlled Voltage Source1/1
  v_abc_ref/1 -> Demux/1
  Demux/2 -> Controlled Voltage Source2/1
  connections:
  Three-Phase Source1/RConn3 -- Subsystem3/LConn6
  Three-Phase Source1/RConn2 -- Subsystem3/LConn5
  Three-Phase Source1/RConn1 -- Subsystem3/LConn4
  Controlled Voltage Source3/RConn1 -- Subsystem3/LConn3
  Controlled Voltage Source2/RConn1 -- Subsystem3/LConn2
  Controlled Voltage Source1/RConn1 -- Subsystem3/LConn1
  Subsystem3/RConn3 -- C/RConn1
  Subsystem3/RConn2 -- B/RConn1
  Subsystem3/RConn1 -- A/RConn1
  Controlled Voltage Source1/LConn1 -- Controlled Voltage Source2/LConn1 -- N/RConn1 -- Three-Phase Source1/LConn1 -- Controlled Voltage Source3/LConn1

== system Sim7_test_var_load/VSC00/Bridge_Model ==
  Uref : Inport
  Constant : Constant
  Memory : Memory
  NOT1 : Logic  Operator=NOT  IconShape=distinctive  AllPortsSameDT=off  OutDataTypeStr=boolean
  Saturation : Saturate  UpperLimit=1  LowerLimit=-1
  Three-Phase Breaker1 : powerlib/Elements/Three-Phase Breaker  InitialState=closed  SwitchA=on  SwitchB=on  SwitchC=on  SwitchTimes="[4/60  10/60]"  External=on  BreakerResistance=0.001  SnubberResistance=1e6  SnubberCapacitance=inf  Measurements=None
  Three-Phase Breaker2 : powerlib/Elements/Three-Phase Breaker  InitialState=open  SwitchA=on  SwitchB=on  SwitchC=on  SwitchTimes="[4/60  10/60]"  External=on  BreakerResistance=0.001  SnubberResistance=1e6  SnubberCapacitance=inf  Measurements=None
  Three-Phase Source : powerlib/Electrical Sources/Three-Phase Source  InternalConnection=Yg  VoltagePhases=off  Voltage=Vvsc0*Un1  PhaseAngle=Theta_vsc0  Voltage_phases=[25e3 25e3 25e3]/sqrt(3)  PhaseAngles_phases=[0 -120 +120]  Frequency=fb  NonIdealSource=off  SpecifyImpedance=off  Resistance=0  Inductance=0  ShortCircuitLevel=100e6  BaseVoltage=VSC01_Un1  XRratio=7  BusType=swing  Pref=0.3  Qref=0  Prefabc=[10e3, 10e3, 10e3]  Qrefabc=[0, 0, 0]  Qmin=-Inf  Qmax=Inf
  Universal Bridge : powerlib/Power Electronics/Universal Bridge  Arms=3  SnubberResistance=1e5  SnubberCapacitance=inf  Device=Average-model based VSC  Ron=1e-3  Lon=0  ForwardVoltages="[  0  0  ]"  ForwardVoltage=0  GTOparameters=[ 10e-6 , 20e-6 ]  IGBTparameters=[ 1e-6 , 2e-6 ]  Measurements=None  Measurements_2=None  converterType=Rectifier
  mp3 : Gain  Gain=2/Udcn
  PhA : PMIOPort  Side=Right
  PhB : PMIOPort  Port=2  Side=Right
  PhC : PMIOPort  Port=3  Side=Right
  Vdc+ : PMIOPort  Port=4  Side=Left
  Vdc- : PMIOPort  Port=5  Side=Left
  wires:
  Saturation/1 -> Universal Bridge/1
  Constant/1 -> Memory/1
  NOT1/1 -> Three-Phase Breaker1/1
  Memory/1 -> NOT1/1, Three-Phase Breaker2/1
  mp3/1 -> Saturation/1
  Uref/1 -> mp3/1
  connections:
  Three-Phase Breaker2/LConn1 -- Three-Phase Breaker1/LConn1 -- PhA/RConn1
  Three-Phase Breaker2/LConn2 -- Three-Phase Breaker1/LConn2 -- PhB/RConn1
  Three-Phase Breaker2/LConn3 -- Three-Phase Breaker1/LConn3 -- PhC/RConn1
  Three-Phase Breaker2/RConn1 -- Universal Bridge/LConn1
  Three-Phase Breaker2/RConn2 -- Universal Bridge/LConn2
  Three-Phase Breaker2/RConn3 -- Universal Bridge/LConn3
  Three-Phase Source/RConn1 -- Three-Phase Breaker1/RConn1
  Three-Phase Source/RConn2 -- Three-Phase Breaker1/RConn2
  Three-Phase Source/RConn3 -- Three-Phase Breaker1/RConn3
  Universal Bridge/RConn1 -- Vdc+/RConn1
  Universal Bridge/RConn2 -- Vdc-/RConn1

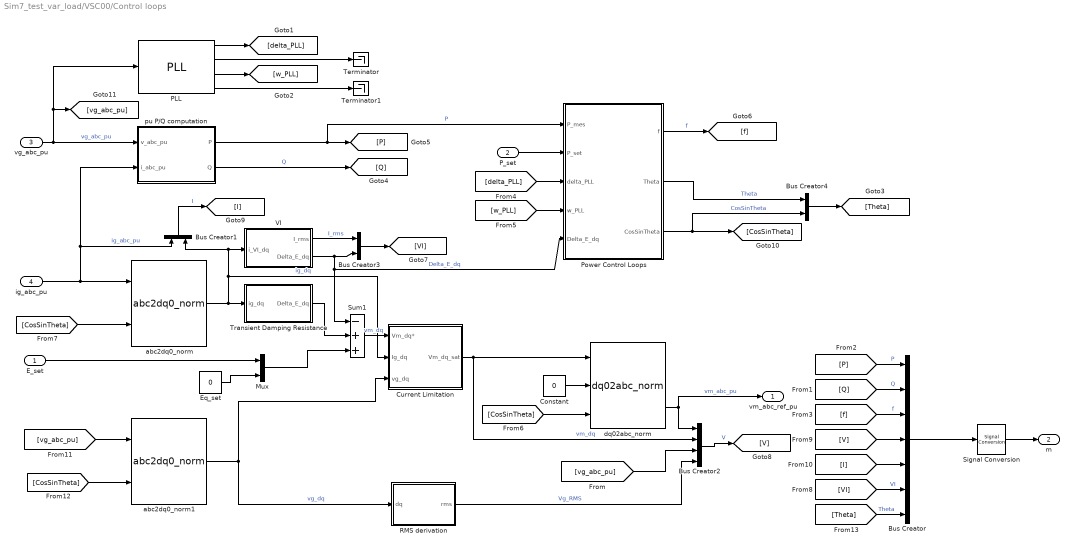
== system Sim7_test_var_load/VSC00/Control loops ==
  E_set : Inport
  P_set : Inport  Port=2
  vg_abc_pu : Inport  Port=3
  ig_abc_pu : Inport  Port=4
  " pu P/Q computation" : Subsystem  DialogController=POWERSYS.PowerSysDialog
  Bus Creator : BusCreator  Inputs=7
  Bus Creator1 : BusCreator  Inputs=2
  Bus Creator2 : BusCreator  Inputs=4
  Bus Creator3 : BusCreator  Inputs=2
  Bus Creator4 : BusCreator  Inputs=2
  Constant : Constant  Value=0
  Current Limitation : Subsystem
  Eq_set : Constant  Value=0
  Mux : Mux  Inputs=2
  PLL : Control_Lib/PLL  fb=fb  Tr_PLL=Tr_PLL  Theta0=Theta0
      settings: SourceProductName=VSC_Lib
  Power Control Loops : Subsystem
  RMS derivation : Subsystem
  Signal Conversion : SignalConversion  OverrideOpt=off
  Sum1 : Sum  Inputs=-++
  Terminator : Terminator
  Terminator1 : Terminator
  Transient Damping Resistance : Subsystem
  VI : Subsystem
  abc2dq0_norm : Control_Lib/abc2dq0_norm  referenceAxisMode=Reference axis at 90 degrees behind phase_a  baseUpdateGain=1/sqrt(3)
      settings: SourceProductName=VSC_Lib
  abc2dq0_norm1 : Control_Lib/abc2dq0_norm  referenceAxisMode=Reference axis at 90 degrees behind phase_a  baseUpdateGain=1/sqrt(3)
      settings: SourceProductName=VSC_Lib
  dq02abc_norm : Control_Lib/dq02abc_norm  referenceAxisMode=Reference axis at 90 degrees behind phase_a  baseUpdateGain=sqrt(3)
      settings: SourceProductName=VSC_Lib
  vm_abc_ref_pu : Outport  VectorParamsAs1DForOutWhenUnconnected=off
  m : Outport  Port=2  VectorParamsAs1DForOutWhenUnconnected=off
  wires:
  [Theta] -> Bus Creator/7  "Theta"
  Bus Creator4/1 -> [Theta]
  RMS derivation/1(rms) -> Bus Creator2/4  "Vg_RMS"
  [vg_abc_pu] -> Bus Creator2/3
  Bus Creator3/1 -> [VI]
  PLL/4 -> Terminator1/1
  PLL/2 -> Terminator/1
  PLL/1 -> [delta_PLL]
  Constant/1 -> dq02abc_norm/2
  Power Control Loops/3(CosSinTheta) -> [CosSinTheta], Bus Creator4/2  "CosSinTheta"
  PLL/3 -> [w_PLL]
  [I] -> Bus Creator/5
  Bus Creator1/1 -> [I]  "I"
  Bus Creator/1 -> Signal Conversion/1
  [VI] -> Bus Creator/6  "VI"
  [V] -> Bus Creator/4
  Bus Creator2/1 -> [V]  "V"
  Eq_set/1 -> Mux/2
  Mux/1 -> Sum1/3
  VI/1(I_rms) -> Bus Creator3/1  "I_rms"
  Transient Damping Resistance/1("Delta_E_dq ") -> Sum1/2
  VI/2(Delta_E_dq) -> Bus Creator3/2, Sum1/1, Power Control Loops/5(Delta_E_dq)  "Delta_E_dq"
  [CosSinTheta] -> abc2dq0_norm/2
  [CosSinTheta] -> dq02abc_norm/3
  Power Control Loops/2(Theta) -> Bus Creator4/1  "Theta"
  abc2dq0_norm/2 -> Bus Creator1/2, VI/1(i_VI_dq), Current Limitation/2(Ig_dq), Transient Damping Resistance/1(ig_dq)  "ig_dq"
  ig_abc_pu/1 -> abc2dq0_norm/1, " pu P/Q computation"/2(i_abc_pu), Bus Creator1/1  "ig_abc_pu"
  " pu P/Q computation"/1(P) -> [P], Power Control Loops/1(P_mes)  "P"
  vg_abc_pu/1 -> PLL/1, [vg_abc_pu], " pu P/Q computation"/1(v_abc_pu)  "vg_abc_pu"
  Power Control Loops/1(f) -> [f]  "f"
  [w_PLL] -> Power Control Loops/4(w_PLL)
  P_set/1 -> Power Control Loops/2(P_set)
  [delta_PLL] -> Power Control Loops/3(delta_PLL)
  Current Limitation/1(Vm_dq_sat) -> dq02abc_norm/1, Bus Creator2/2  "vm_dq"
  " pu P/Q computation"/2(Q) -> [Q]  "Q"
  E_set/1 -> Mux/1
  dq02abc_norm/2 -> Bus Creator2/1, vm_abc_ref_pu/1  "vm_abc_pu"
  [f] -> Bus Creator/3  "f"
  [Q] -> Bus Creator/2  "Q"
  [P] -> Bus Creator/1  "P"
  Signal Conversion/1 -> m/1
  Sum1/1 -> Current Limitation/1(Vm_dq*)  "vm_dq"
  [vg_abc_pu] -> abc2dq0_norm1/1
  [CosSinTheta] -> abc2dq0_norm1/2
  abc2dq0_norm1/2 -> Current Limitation/3(vg_dq), RMS derivation/1(dq)  "vg_dq"

== system Sim7_test_var_load/Infinite_Grid/InertialDqVoltageSource/NetworkLeadLagTimeConstants ==
  In1 : Inport
  Integrator3 : Integrator  InitialCondition=(P0/Sb)*(1-TN/TD)
  Sum1 : Sum
  Sum2 : Sum  Inputs=+-
  mp1 : Gain  Gain=TN/TD
  mp2 : Gain  Gain=1-TN/TD
  mp3 : Gain  Gain=1/TD
  Out1 : Outport  VectorParamsAs1DForOutWhenUnconnected=off
  wires:
  Sum2/1 -> mp3/1
  mp3/1 -> Integrator3/1
  Integrator3/1 -> Sum1/2, Sum2/2
  In1/1 -> mp1/1, mp2/1
  mp2/1 -> Sum2/1
  mp1/1 -> Sum1/1
  Sum1/1 -> Out1/1

== system Sim7_test_var_load/Infinite_Grid/Source_For_OP/Subsystem3 ==
  switch : Inport
  Breaker : powerlib/Elements/Breaker  InitialState=0  SwitchingTimes="[1/60  5/60]"  External=on  BreakerResistance=0.001  SnubberResistance=1e6  SnubberCapacitance=inf  Measurements=None  MoreParameters=on  NoBreakLoop=off
  Breaker1 : powerlib/Elements/Breaker  InitialState=0  SwitchingTimes="[1/60  5/60]"  External=on  BreakerResistance=0.001  SnubberResistance=1e6  SnubberCapacitance=inf  Measurements=None  MoreParameters=on  NoBreakLoop=off
  Breaker2 : powerlib/Elements/Breaker  InitialState=0  SwitchingTimes="[1/60  5/60]"  External=on  BreakerResistance=0.001  SnubberResistance=1e6  SnubberCapacitance=inf  Measurements=None  MoreParameters=on  NoBreakLoop=off
  Breaker3 : powerlib/Elements/Breaker  InitialState=1  SwitchingTimes="[1/60  5/60]"  External=on  BreakerResistance=0.001  SnubberResistance=1e6  SnubberCapacitance=inf  Measurements=None  MoreParameters=on  NoBreakLoop=off
  Breaker4 : powerlib/Elements/Breaker  InitialState=1  SwitchingTimes="[1/60  5/60]"  External=on  BreakerResistance=0.001  SnubberResistance=1e6  SnubberCapacitance=inf  Measurements=None  MoreParameters=on  NoBreakLoop=off
  Breaker5 : powerlib/Elements/Breaker  InitialState=1  SwitchingTimes="[1/60  5/60]"  External=on  BreakerResistance=0.001  SnubberResistance=1e6  SnubberCapacitance=inf  Measurements=None  MoreParameters=on  NoBreakLoop=off
  Logical Operator : Logic  Operator=NOT  AllPortsSameDT=off  OutDataTypeStr=boolean
  A : PMIOPort  Side=Left
  B : PMIOPort  Port=2  Side=Left
  C : PMIOPort  Port=3  Side=Left
  Ainit : PMIOPort  Port=4  Side=Left
  Binit : PMIOPort  Port=5  Side=Left
  Cinit : PMIOPort  Port=6  Side=Left
  a : PMIOPort  Port=7  Side=Right
  b : PMIOPort  Port=8  Side=Right
  c : PMIOPort  Port=9  Side=Right
  wires:
  Logical Operator/1 -> Breaker3/1, Breaker4/1, Breaker5/1
  switch/1 -> Logical Operator/1, Breaker/1, Breaker1/1, Breaker2/1
  connections:
  Breaker4/RConn1 -- Breaker1/RConn1 -- b/RConn1
  a/RConn1 -- Breaker3/RConn1 -- Breaker/RConn1
  Breaker1/LConn1 -- B/RConn1
  Breaker3/LConn1 -- Ainit/RConn1
  Breaker2/LConn1 -- C/RConn1
  Breaker4/LConn1 -- Binit/RConn1
  Breaker2/RConn1 -- Breaker5/RConn1 -- c/RConn1
  Breaker5/LConn1 -- Cinit/RConn1
  Breaker/LConn1 -- A/RConn1

== system Sim7_test_var_load/VSC00/Control loops/ pu P//Q computation ==
  v_abc_pu : Inport  PortDimensions=3
  i_abc_pu : Inport  Port=2  PortDimensions=3
  Demux : Demux  Outputs=3
      settings: DisplayOption=none
  Mux : Mux  Inputs=3
  Product1 : Product  InputSameDT=on  SaturateOnIntegerOverflow=on  OutDataTypeStr=Inherit: Same as first input
  Product3 : Product  InputSameDT=on  SaturateOnIntegerOverflow=on  OutDataTypeStr=Inherit: Same as first input
  Sum : Sum  Inputs=+-  InputSameDT=on  SaturateOnIntegerOverflow=on  OutDataTypeStr=Inherit: Same as first input
  Sum1 : Sum  Inputs=1  InputSameDT=on  SaturateOnIntegerOverflow=on  OutDataTypeStr=Inherit: Same as first input
  Sum4 : Sum  Inputs=1  InputSameDT=on  SaturateOnIntegerOverflow=on  OutDataTypeStr=Inherit: Same as first input
  Sum5 : Sum  Inputs=+-  InputSameDT=on  SaturateOnIntegerOverflow=on  OutDataTypeStr=Inherit: Same as first input
  Sum6 : Sum  Inputs=+-  InputSameDT=on  SaturateOnIntegerOverflow=on  OutDataTypeStr=Inherit: Same as first input
  pu->V : Gain  Gain=1/sqrt(3)  SaturateOnIntegerOverflow=on  OutDataTypeStr=Inherit: Same as input  ParamDataTypeStr=Inherit: Same as input
  pu->V1 : Gain  Gain=1/3  SaturateOnIntegerOverflow=on  OutDataTypeStr=Inherit: Same as input  ParamDataTypeStr=Inherit: Same as input
  pu->V2 : Gain  Gain=1/3  SaturateOnIntegerOverflow=on  OutDataTypeStr=Inherit: Same as input  ParamDataTypeStr=Inherit: Same as input
  P : Outport  VectorParamsAs1DForOutWhenUnconnected=off
  Q : Outport  Port=2  VectorParamsAs1DForOutWhenUnconnected=off
  wires:
  pu->V2/1 -> Q/1
  pu->V1/1 -> P/1
  Sum1/1 -> pu->V/1
  Product3/1 -> Sum1/1
  Product1/1 -> Sum4/1
  v_abc_pu/1 -> Product1/1, Demux/1
  i_abc_pu/1 -> Product1/2, Product3/2
  Sum4/1 -> pu->V1/1
  Demux/1 -> Sum/1, Sum6/2
  Demux/2 -> Sum/2, Sum5/1
  Demux/3 -> Sum5/2, Sum6/1
  Sum/1 -> Mux/3
  Sum5/1 -> Mux/1
  Sum6/1 -> Mux/2
  Mux/1 -> Product3/1
  pu->V/1 -> pu->V2/1  "Q"
